simulink model "Geometric_Control"  (R2023a)
settings: Solver=VariableStepAuto  StartTime=0.0  StopTime=T  RelTol=1e-3
InitFcn:
  | %% INITIALIZATION
  | run('LOAD_GEOMETRIC.m');
  | mass = 0.85;
  | Ib = diag([2.5 2.1 4.3])*10^-2;
  | %% SAMPLING TIME
  | Ts=0.001;
values from neighbouring files (symbols this model uses):
  PP = [-1 -1.2 2 0 -0.999982179716 -1.19999407978 1.99999992207 0.01 -0.999859649731 -1.19995305914 1.99999937818 0.02 ... (16004 elements, 4x4001)]    [POS_40.mat]
libraries: robotcorelib x1, uavutilslib x1
settings Model: Creator=salvatoregranata  LastModifiedBy=salvatoregranata

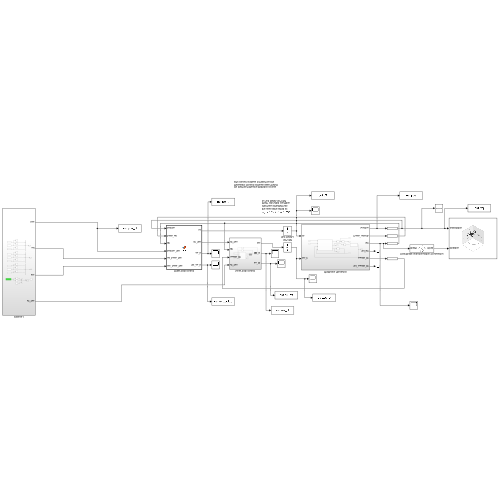
[thumbnail: Simulink's stored preview of the top-level diagram]
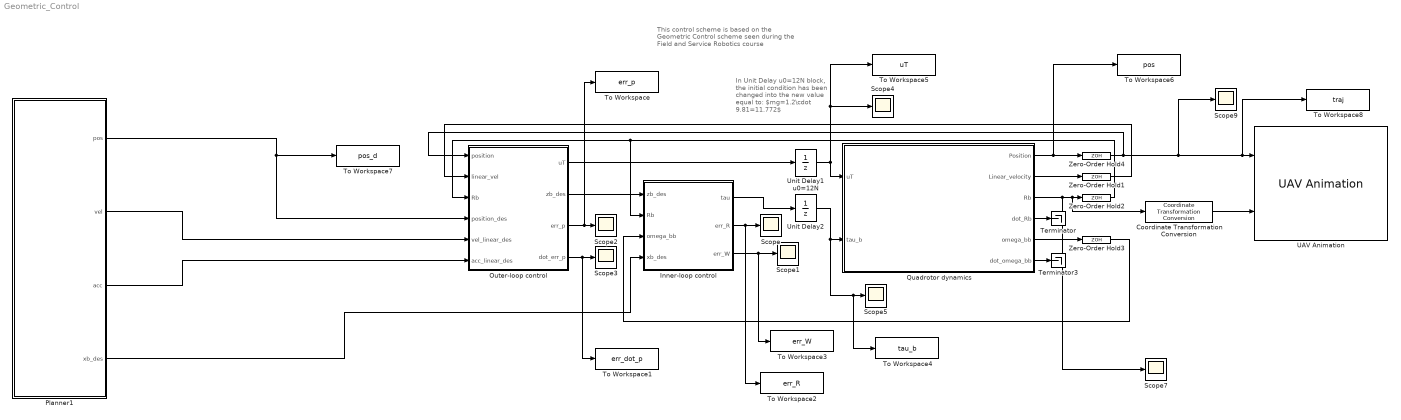
== system Geometric_Control ==
  note: This control scheme is based on the Geometric Control scheme seen during the Field and Service Robotics course
  note: In Unit Delay u0=12N block, the initial condition has been changed into the new value equal to: $mg=1.2\cdot 9.81=11.772$
  Coordinate Transformation Conversion : robotcorelib/Coordinate Transformation Conversion  InputRepresentation=Rotation Matrix  InputEulerSequence=ZYX  ShowTrVecInputPort=on  OutputRepresentation=Quaternion  OutputEulerSequence=ZYX  ShowTrVecOutputPort=on  SimulateUsing=Interpreted execution
  Inner-loop control : Subsystem
  Outer-loop control : MATLAB Function  TreatAsAtomicUnit=on
  Planner1 : Subsystem
  Quadrotor dynamics : Subsystem
  Scope{,1..5,7,9} (8 alike) : Scope
  Terminator : Terminator
  Terminator3 : Terminator
  To Workspace : ToWorkspace  VariableName=err_p  SaveFormat=Structure With Time  SampleTime=-1
  To Workspace1 : ToWorkspace  VariableName=err_dot_p  SaveFormat=Structure With Time  SampleTime=-1
  To Workspace2 : ToWorkspace  VariableName=err_R  SaveFormat=Structure With Time  SampleTime=-1
  To Workspace3 : ToWorkspace  VariableName=err_W  SaveFormat=Structure With Time  SampleTime=-1
  To Workspace4 : ToWorkspace  VariableName=tau_b  SaveFormat=Structure With Time  SampleTime=-1
  To Workspace5 : ToWorkspace  VariableName=uT  SaveFormat=Structure With Time  SampleTime=-1
  To Workspace6 : ToWorkspace  VariableName=pos  SaveFormat=Structure With Time  SampleTime=-1
  To Workspace7 : ToWorkspace  VariableName=pos_d  SaveFormat=Structure With Time  SampleTime=-1
  To Workspace8 : ToWorkspace  VariableName=traj  SaveFormat=Structure With Time  SampleTime=-1
  UAV Animation : uavutilslib/UAV Animation  UAVType=Multirotor  UAVSize=1  InertialZDirection=Up  SampleTime=0.1
  Unit Delay1 u0=12N : UnitDelay  InitialCondition=11.772  SampleTime=Ts
  Unit Delay2 : UnitDelay  InitialCondition=[0 0 0]  SampleTime=Ts
  Zero-Order Hold{1..4} (4 alike) : ZeroOrderHold  SampleTime=Ts
  wires:
  Outer-loop control/3(err_p) -> To Workspace/1, Scope2/1
  Outer-loop control/2(zb_des) -> Inner-loop control/1(zb_des)
  Zero-Order Hold3/1 -> Inner-loop control/3(omega_bb)
  Zero-Order Hold1/1 -> Outer-loop control/2(linear_vel)
  Coordinate Transformation Conversion/1 -> UAV Animation/2
  Planner1/4(xb_des) -> Inner-loop control/4(xb_des)
  Zero-Order Hold2/1 -> Outer-loop control/3(Rb), Inner-loop control/2(Rb)
  Unit Delay1 u0=12N/1 -> Quadrotor dynamics/1(uT), To Workspace5/1, Scope4/1
  Outer-loop control/4(dot_err_p) -> To Workspace1/1, Scope3/1
  Quadrotor dynamics/1(Position) -> To Workspace6/1, Zero-Order Hold4/1
  Quadrotor dynamics/4(dot_Rb) -> Terminator/1
  Unit Delay2/1 -> To Workspace4/1, Scope5/1, Quadrotor dynamics/2(tau_b)
  Quadrotor dynamics/2(Linear_velocity) -> Zero-Order Hold1/1
  Planner1/1(pos) -> Outer-loop control/4(position_des), To Workspace7/1
  Planner1/3(acc) -> Outer-loop control/6(acc_linear_des)
  Planner1/2(vel) -> Outer-loop control/5(vel_linear_des)
  Quadrotor dynamics/6(dot_omega_bb) -> Terminator3/1
  Quadrotor dynamics/5(omega_bb) -> Zero-Order Hold3/1
  Outer-loop control/1(uT) -> Unit Delay1 u0=12N/1
  Inner-loop control/2(err_R) -> To Workspace2/1, Scope/1
  Zero-Order Hold4/1 -> Scope9/1, To Workspace8/1, UAV Animation/1, Outer-loop control/1(position)
  Quadrotor dynamics/3(Rb) -> Coordinate Transformation Conversion/1, Zero-Order Hold2/1, Scope7/1
  Inner-loop control/1(tau) -> Unit Delay2/1
  Inner-loop control/3(err_W) -> To Workspace3/1, Scope1/1

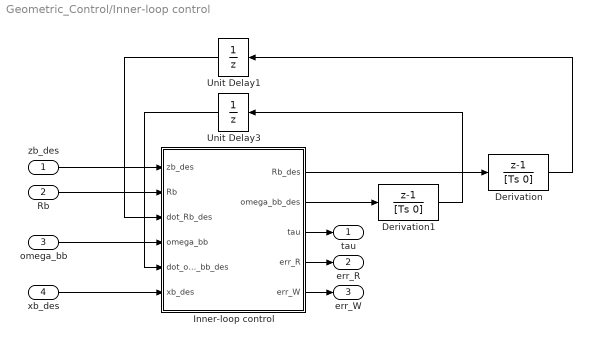
== system Geometric_Control/Inner-loop control ==
  zb_des : Inport
  Rb : Inport  Port=2
  omega_bb : Inport  Port=3
  xb_des : Inport  Port=4
  Derivation : DiscreteTransferFcn  Numerator=[1 -1]  Denominator=[Ts 0]  InitialStates=[1 0 0;0 1 0;0 0 1]  SampleTime=Ts
  Derivation1 : DiscreteTransferFcn  Numerator=[1 -1]  Denominator=[Ts 0]  InitialStates=[0 0 0]  SampleTime=Ts
  Inner-loop control : MATLAB Function  TreatAsAtomicUnit=on
  Unit Delay1 : UnitDelay  InitialCondition=eye(3)  SampleTime=Ts
  Unit Delay3 : UnitDelay  InitialCondition=[0 0 0]  SampleTime=Ts
  tau : Outport
  err_R : Outport  Port=2
  err_W : Outport  Port=3
  wires:
  xb_des/1 -> Inner-loop control/6(xb_des)
  Inner-loop control/4(err_R) -> err_R/1
  Rb/1 -> Inner-loop control/2(Rb)
  Inner-loop control/3(tau) -> tau/1
  Unit Delay1/1 -> Inner-loop control/3(dot_Rb_des)
  Derivation1/1 -> Unit Delay3/1
  Inner-loop control/5(err_W) -> err_W/1
  Unit Delay3/1 -> Inner-loop control/5(dot_omega_bb_des)
  Derivation/1 -> Unit Delay1/1
  zb_des/1 -> Inner-loop control/1(zb_des)
  omega_bb/1 -> Inner-loop control/4(omega_bb)
  Inner-loop control/1(Rb_des) -> Derivation/1
  Inner-loop control/2(omega_bb_des) -> Derivation1/1

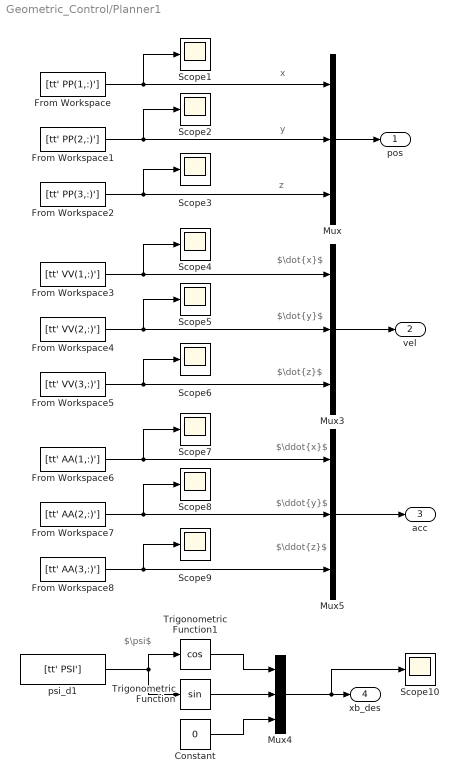
== system Geometric_Control/Planner1 ==
  note: $\psi$
  note: $\dot{x}$
  note: x
  note: y
  note: z
  note: $\dot{y}$
  note: $\dot{z}$
  note: $\ddot{z}$
  note: $\ddot{y}$
  note: $\ddot{x}$
  Constant : Constant  Value=0
  From Workspace : FromWorkspace  VariableName=[tt' PP(1,:)']
  From Workspace1 : FromWorkspace  VariableName=[tt' PP(2,:)']
  From Workspace2 : FromWorkspace  VariableName=[tt' PP(3,:)']
  From Workspace3 : FromWorkspace  VariableName=[tt' VV(1,:)']
  From Workspace4 : FromWorkspace  VariableName=[tt' VV(2,:)']
  From Workspace5 : FromWorkspace  VariableName=[tt' VV(3,:)']
  From Workspace6 : FromWorkspace  VariableName=[tt' AA(1,:)']
  From Workspace7 : FromWorkspace  VariableName=[tt' AA(2,:)']
  From Workspace8 : FromWorkspace  VariableName=[tt' AA(3,:)']
  Mux{,3..5} (4 alike) : Mux  Inputs=3
  Scope{1..10} (10 alike) : Scope
  Trigonometric Function : Trigonometry
  Trigonometric Function1 : Trigonometry  Operator=cos
  psi_d1 : FromWorkspace  VariableName=[tt' PSI']  SampleTime=Ts
  pos : Outport
  vel : Outport  Port=2
  acc : Outport  Port=3
  xb_des : Outport  Port=4
  wires:
  Mux5/1 -> acc/1
  From Workspace1/1 -> Mux/2, Scope2/1
  Mux3/1 -> vel/1
  From Workspace6/1 -> Mux5/1, Scope7/1
  From Workspace2/1 -> Mux/3, Scope3/1
  From Workspace4/1 -> Mux3/2, Scope5/1
  Mux/1 -> pos/1
  From Workspace/1 -> Mux/1, Scope1/1
  From Workspace7/1 -> Mux5/2, Scope8/1
  From Workspace8/1 -> Mux5/3, Scope9/1
  From Workspace3/1 -> Mux3/1, Scope4/1
  From Workspace5/1 -> Mux3/3, Scope6/1
  Trigonometric Function1/1 -> Mux4/1
  Trigonometric Function/1 -> Mux4/2
  Constant/1 -> Mux4/3
  psi_d1/1 -> Trigonometric Function/1, Trigonometric Function1/1
  Mux4/1 -> Scope10/1, xb_des/1

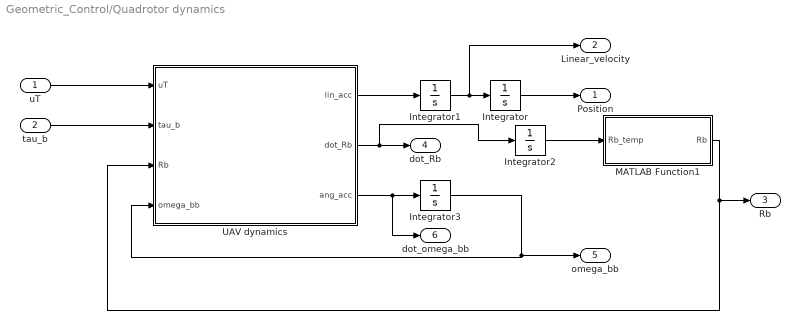
== system Geometric_Control/Quadrotor dynamics ==
  uT : Inport
  tau_b : Inport  Port=2
  Integrator : Integrator  InitialCondition=[PP(1,1) PP(2,1) PP(3,1)]
  Integrator1 : Integrator  InitialCondition=[0 0 0]
  Integrator2 : Integrator  InitialCondition=[1 0 0; 0 1 0;0 0 1]
  Integrator3 : Integrator  InitialCondition=[0 0 0]
  MATLAB Function1 : MATLAB Function  TreatAsAtomicUnit=on
  UAV dynamics : MATLAB Function  TreatAsAtomicUnit=on
  Position : Outport
  Linear_velocity : Outport  Port=2
  Rb : Outport  Port=3
  dot_Rb : Outport  Port=4
  omega_bb : Outport  Port=5
  dot_omega_bb : Outport  Port=6
  wires:
  tau_b/1 -> UAV dynamics/2(tau_b)
  Integrator/1 -> Position/1
  UAV dynamics/3(ang_acc) -> dot_omega_bb/1, Integrator3/1
  UAV dynamics/1(lin_acc) -> Integrator1/1
  uT/1 -> UAV dynamics/1(uT)
  Integrator1/1 -> Linear_velocity/1, Integrator/1
  Integrator3/1 -> UAV dynamics/4(omega_bb), omega_bb/1
  UAV dynamics/2(dot_Rb) -> Integrator2/1, dot_Rb/1
  MATLAB Function1/1(Rb) -> Rb/1, UAV dynamics/3(Rb)
  Integrator2/1 -> MATLAB Function1/1(Rb_temp)

== matlab function Geometric_Control/Quadrotor dynamics/UAV dynamics ==
  data: uT input size=1; tau_b input size=3; lin_acc output size=3; Rb input size=[3,3]; omega_bb input size=3; dot_Rb output size=[3,3]; ang_acc output size=3; mass parameter size=1; Ib parameter size=[3,3]
function [lin_acc, dot_Rb, ang_acc] = fcn(uT,tau_b,Rb,omega_bb,mass, Ib)

lin_acc = 9.81*[0 0 1]'-(uT/mass)*Rb*[0 0 1]';
dot_Rb = Rb*skew(omega_bb);
ang_acc = inv(Ib)*(-skew(omega_bb)*Ib*omega_bb + tau_b);

end

function S = skew(v)
if(numel(v)~= 1)
S= [0 -v(3) v(2); 
    v(3) 0 -v(1);
    -v(2) v(1) 0];
else
S= zeros(3);
end
end

== matlab function Geometric_Control/Outer-loop control ==
  data: position input size=3; uT output size=1; linear_vel input size=3; Rb input size=[3,3]; zb_des output size=3; mass parameter size=1; position_des input size=3; vel_linear_des input size=3; acc_linear_des input size=3; err_p output size=3; dot_err_p output size=3
function [uT, zb_des, err_p, dot_err_p] = fcn(position, linear_vel, Rb, mass, ...
    position_des, vel_linear_des, acc_linear_des)


e3=[0 0 1]';
Kp=diag([10 10 20]);
Kv=diag([2 2 5]);
g=9.81;

err_p=position-position_des;

dot_err_p=linear_vel-vel_linear_des;

uT=-(-Kp*err_p-Kv*dot_err_p-mass*g*e3+mass*acc_linear_des)'* Rb*e3;

zb_des=-(-Kp*err_p-Kv*dot_err_p-mass*g*e3+mass*acc_linear_des)/norm(-Kp*err_p-Kv*dot_err_p-mass*g*e3+mass*acc_linear_des);

== matlab function Geometric_Control/Inner-loop control/Inner-loop control ==
  data: Rb_des output size=[3,3]; omega_bb_des output size=3; tau output size=3; zb_des input size=3; Rb input size=[3,3]; dot_Rb_des input size=[3,3]; omega_bb input size=3; dot_omega_bb_des input size=3; xb_des input size=3; Ib parameter size=[3,3]; err_R output size=3; err_W output size=3
function [Rb_des, omega_bb_des, tau, err_R, err_W] = fcn(zb_des, Rb, dot_Rb_des, omega_bb, dot_omega_bb_des, xb_des, Ib)

yb_des=skew(zb_des)*xb_des/norm(skew(zb_des)*xb_des);
Rb_des=[skew(yb_des)*zb_des, yb_des,zb_des];

omega_bb_des = wedge(Rb_des'*dot_Rb_des);

err_R=wedge(Rb_des'*Rb-Rb'*Rb_des)/2;
err_W=omega_bb-Rb'*Rb_des*omega_bb_des;


Kr=diag([10 10 20]);
Kw=diag([3 3 7]);
tau=-Kr*err_R-Kw*err_W+skew(omega_bb)*Ib*omega_bb-Ib*(skew(omega_bb)*Rb'*Rb_des*omega_bb_des-Rb'*Rb_des*dot_omega_bb_des);

end

function S = skew(v)
if(numel(v)~= 1)
S= [0 -v(3) v(2); 
    v(3) 0 -v(1);
    -v(2) v(1) 0];
else
S= zeros(3);
end
end

function v = wedge(S)
v1 = S(3,2);
v2 = S(1,3);
v3 = S(2,1);
v = [v1 v2 v3]';
end

== matlab function Geometric_Control/Quadrotor dynamics/MATLAB Function1 ==
  data: Rb_temp input; Rb output
function Rb = fcn(Rb_temp)
    [U,S,V] = svd(Rb_temp);
    sigma = det(U*V');
    S_ = diag([1 1 sigma]);

    Rb = U*S_*V';
end
